simulink model "vasastaden_sort"  (Simulink 5.0)
settings: Solver=FixedStepDiscrete  SolverMode=SingleTasking  StartTime=0  StopTime=Q  FixedStep=1  RelTol=1e-3
values from neighbouring files (symbols this model uses):
  andpt = 1/3    (= 0.333333333333)    [constants_trafik.m]
  andt = 0.1    [constants_trafik.m]
  baseflow = str2num(get(HH, 'String'))    [inputs.m]
  baseflow2 = 0    [areas2.m]
  delayinit = [zeros(1,nr_ex_H2O)]    [constants_trafik.m]
  fast = 0.7    [constants_trafik.m]
  fkmday = in_fkmday    [areas.m]
  fkmday2 = 32067    [areas2.m]
  init_init = 4*3600    (= 14400)    [areas.m]
  init_time = 5    [areas.m]
  K2 = 0.03    [areas2.m]
  nhv = in_nhv/100    [areas.m]
  nhv2 = 5/100    (= 0.05)    [areas2.m]
  nr_ex_H2O = totnr-1    (= 20)    [Prep.m]
  numberOfPersons = in_numberOfPersons    [Prep.m]
  numberOfPersons2 = 5115    [areas2.m]
  othera = in_otherarea    [areas.m]
  othera2 = 42282    [areas2.m]
  othermax = drydepmax*othera    [constants_trafik.m]
  othermax2 = drydepmax*othera2    [areas2.m]
  redu = 0.8    [areas.m]
  roada = in_roads    [areas.m]
  roada2 = 95962    [areas2.m]
  roadaccmax = dryper*24*sph*fast*(p_tyrewear+p_roadwear+p_exhaust+p_breakwear+p_drydep+p_corrZn+p_oildischarge+p_catalyst)    [constants_trafik.m]
  roadaccmax2 = dryper*24*sph*fast*(p_tyrewear2+p_roadwear2+p_exhaust2+p_breakwear2+p_drydep2+p_corrZn2+p_oildischarge2+p_catalyst2)    [areas2.m]
  roadkm = 67e9    (= 67000000000)    [constants_trafik.m]
  roadrunpart = 1    [constants_trafik.m]
  roadwear = 130000    [constants_trafik.m]
  roadZna = in_part_roadZna/100*roada    [areas.m]
  roadZna2 = 2/100*roada2    (= 1919.24)    [areas2.m]
  roofa = in_roofs    [areas.m]
  roofa2 = 92958    [areas2.m]
  RoofCua = in_part_roofCua/100*roofa/cos(15*pi/180)    [areas.m]
  RoofCua2 = 6.9/100*roofa2/cos(15*pi/180)    [areas2.m]
  roofmax = (Znroofmax*RoofZna+Curoofmax*RoofCua)*roofrunpart+drydepmax*roofa    [constants_trafik.m]
  roofmax2 = (Znroofmax*RoofZna2+Curoofmax*RoofCua2)*roofrunpart+drydepmax*roofa2    [areas2.m]
  roofrunpart = 0.7    [constants_trafik.m]
  RoofZna = in_part_roofZna/100*roofa/cos(15*pi/180)    [areas.m]
  RoofZna2 = 6.4/100*roofa2/cos(15*pi/180)    [areas2.m]
  sec_per_ts = in_sec_per_ts    [Prep.m]
  sph = 3600/sec_per_ts    [Prep.m]
  tota = in_tota    [areas.m]
  totnr = 21    [Prep.m]
  tyrewear = 9000    [constants_trafik.m]
  wetdep = [sum(s_wetdep(:,i))]*tota*trans1    [polldistr_gr.m]
  yearly_rain = 1    [Callback_simulate.m]    (also in SEWSYS_fig.m)
undefined symbols (not defined in the file or in its folder): BDT, BODofVS, brakep, catalystp, Curoofp, Drainage, drydep, exhp, Faeces, Industry, K, K2r, oilp, ProcSS_bio, ProcSS_chem, ProcSS_presed, ProcSS_sand, ProcSS_screen, roadp, sani, spBiooxidBod, spBiored, spCcontent, spChemFe, spChemicalPart, spCODBOD, spDenSS, spHeavym, spHjust, spN2ONpurEmitted, spNemitted, spNitrif, spNpur, spOcontent, spPBound, spPout, spPout1, spVSofSS, SSred_bio, SSred_chem, SSred_presed, SSred_sand, SSred_screen, SStoWater, stormw, tyrep, Urine, VSofSS_sand, VSofSS_screen, Znroofp
libraries: SEWSYS_library x1
(part 2 of 3)

== system vasastaden_sort/Sewage plant/Pre-sedimentation/Separation/3-6 ==
  in_1 : Inport  Orientation=down
  "in_2 " : Inport  Orientation=down  Port=2
  Ground1 : Ground  Orientation=down
  Mux : Mux  Orientation=down
  N-tot : MATLABFcn  Orientation=down  MATLABFcn=(u(1)-u(2)-u(3))*SSred_presed  OutputDimensions=1
  NH4 : Product  Orientation=down  SaturateOnIntegerOverflow=on  InputSameDT=on
  "NH4 " : Fcn  Orientation=down  Expr=u(2)
  NH5 : Product  Orientation=down  SaturateOnIntegerOverflow=on  InputSameDT=on
  NO3 : Fcn  Orientation=down  Expr=u(3)
  Sum : Sum  Orientation=down  Inputs=+++  SaturateOnIntegerOverflow=on  InputSameDT=on
  out_1 : Outport  Orientation=down  InitialOutput=0
  wires:
  NH4/1 -> Mux/2, Sum/2
  in_1/1 -> NH5/1, NH4/1
  Mux/1 -> out_1/1
  N-tot/1 -> Sum/1
  Sum/1 -> Mux/1
  "NH4 "/1 -> NH4/2
  NO3/1 -> NH5/2
  "in_2 "/1 -> NO3/1, "NH4 "/1, N-tot/1
  NH5/1 -> Sum/3, Mux/3
  Ground1/1 -> Mux/4

== system vasastaden_sort/Sewage plant/Pre-sedimentation/Separation/if u>0 then 1/u else 0 ==
  note: if u<=0, 0, else 1/u, end
  in_1 : Inport  Orientation=left
  Constant : Constant  Orientation=left  Value=0
  Constant1 : Constant  Orientation=left
  Switch : Switch  Orientation=left  SaturateOnIntegerOverflow=on  InputSameDT=on
  Switch1 : Switch  Orientation=left  SaturateOnIntegerOverflow=on  InputSameDT=on
  inv. : Fcn  Orientation=left  Expr=1/u
  neg : Gain  Orientation=left  Gain=-1  SaturateOnIntegerOverflow=on
  neg1 : Gain  Orientation=left  Gain=-1  SaturateOnIntegerOverflow=on
  out_1 : Outport  Orientation=left  InitialOutput=0
  wires:
  Constant/1 -> Switch/1
  neg/1 -> Switch/2
  Switch/1 -> out_1/1
  inv./1 -> Switch/3
  Switch1/1 -> inv./1
  neg1/1 -> Switch1/2
  Constant1/1 -> Switch1/1
  in_1/1 -> neg/1, neg1/1, Switch1/3

== system vasastaden_sort/Sewage plant/Pre-sedimentation/spVSofSS/if u>0 then 1/u else 0 ==
  note: if u<=0, 0, else 1/u, end
  in_1 : Inport  Orientation=left
  Constant : Constant  Orientation=left  Value=0
  Constant1 : Constant  Orientation=left
  Switch : Switch  Orientation=left  SaturateOnIntegerOverflow=on  InputSameDT=on
  Switch1 : Switch  Orientation=left  SaturateOnIntegerOverflow=on  InputSameDT=on
  inv. : Fcn  Orientation=left  Expr=1/u
  neg : Gain  Orientation=left  Gain=-1  SaturateOnIntegerOverflow=on
  neg1 : Gain  Orientation=left  Gain=-1  SaturateOnIntegerOverflow=on
  out_1 : Outport  Orientation=left  InitialOutput=0
  wires:
  inv./1 -> Switch/3
  Constant/1 -> Switch/1
  neg/1 -> Switch/2
  Switch1/1 -> inv./1
  Switch/1 -> out_1/1
  neg1/1 -> Switch1/2
  Constant1/1 -> Switch1/1
  in_1/1 -> neg/1, neg1/1, Switch1/3

== system vasastaden_sort/Sewage plant/Sandpit/Separation/3-6 ==
  in_1 : Inport  Orientation=down
  "in_2 " : Inport  Orientation=down  Port=2
  Ground2 : Ground  Orientation=down
  Mux : Mux  Orientation=down
  N-tot : MATLABFcn  Orientation=down  MATLABFcn=(u(1)-u(2)-u(3))*SSred_sand  OutputDimensions=1
  NH4 : Product  Orientation=down  SaturateOnIntegerOverflow=on  InputSameDT=on
  "NH4 " : Fcn  Orientation=down  Expr=u(2)
  NH5 : Product  Orientation=down  SaturateOnIntegerOverflow=on  InputSameDT=on
  NO3 : Fcn  Orientation=down  Expr=u(3)
  Sum : Sum  Orientation=down  Inputs=+++  SaturateOnIntegerOverflow=on  InputSameDT=on
  out_1 : Outport  Orientation=down  InitialOutput=0
  wires:
  Ground2/1 -> Mux/4
  NH5/1 -> Mux/3, Sum/3
  "in_2 "/1 -> N-tot/1, "NH4 "/1, NO3/1
  NO3/1 -> NH5/2
  "NH4 "/1 -> NH4/2
  Sum/1 -> Mux/1
  N-tot/1 -> Sum/1
  Mux/1 -> out_1/1
  in_1/1 -> NH4/1, NH5/1
  NH4/1 -> Sum/2, Mux/2

== system vasastaden_sort/Sewage plant/Sandpit/Separation/if u>0 then 1/u else 0 ==
  note: if u<=0, 0, else 1/u, end
  in_1 : Inport  Orientation=left
  Constant : Constant  Orientation=left  Value=0
  Constant1 : Constant  Orientation=left
  Switch : Switch  Orientation=left  SaturateOnIntegerOverflow=on  InputSameDT=on
  Switch1 : Switch  Orientation=left  SaturateOnIntegerOverflow=on  InputSameDT=on
  inv. : Fcn  Orientation=left  Expr=1/u
  neg : Gain  Orientation=left  Gain=-1  SaturateOnIntegerOverflow=on
  neg1 : Gain  Orientation=left  Gain=-1  SaturateOnIntegerOverflow=on
  out_1 : Outport  Orientation=left  InitialOutput=0
  wires:
  Switch/1 -> out_1/1
  neg/1 -> Switch/2
  Constant/1 -> Switch/1
  inv./1 -> Switch/3
  Switch1/1 -> inv./1
  neg1/1 -> Switch1/2
  Constant1/1 -> Switch1/1
  in_1/1 -> neg/1, neg1/1, Switch1/3

== system vasastaden_sort/Sewage plant/Screen/Separation/3-6 ==
  in_1 : Inport  Orientation=down
  "in_2 " : Inport  Orientation=down  Port=2
  Ground : Ground  Orientation=down
  Mux : Mux  Orientation=down
  N-tot : MATLABFcn  Orientation=down  MATLABFcn=(u(1)-u(2)-u(3))*SSred_screen  OutputDimensions=1
  NH4 : Product  Orientation=down  SaturateOnIntegerOverflow=on  InputSameDT=on
  "NH4 " : Fcn  Orientation=down  Expr=u(2)
  NH5 : Product  Orientation=down  SaturateOnIntegerOverflow=on  InputSameDT=on
  NO3 : Fcn  Orientation=down  Expr=u(3)
  Sum : Sum  Orientation=down  Inputs=+++  SaturateOnIntegerOverflow=on  InputSameDT=on
  out_1 : Outport  Orientation=down  InitialOutput=0
  wires:
  NH4/1 -> Mux/2, Sum/2
  in_1/1 -> NH5/1, NH4/1
  Mux/1 -> out_1/1
  N-tot/1 -> Sum/1
  Sum/1 -> Mux/1
  "NH4 "/1 -> NH4/2
  NO3/1 -> NH5/2
  "in_2 "/1 -> NO3/1, "NH4 "/1, N-tot/1
  NH5/1 -> Sum/3, Mux/3
  Ground/1 -> Mux/4

== system vasastaden_sort/Sewage plant/Screen/Separation/if u>0 then 1/u else 0 ==
  note: if u<=0, 0, else 1/u, end
  in_1 : Inport  Orientation=left
  Constant : Constant  Orientation=left  Value=0
  Constant1 : Constant  Orientation=left
  Switch : Switch  Orientation=left  SaturateOnIntegerOverflow=on  InputSameDT=on
  Switch1 : Switch  Orientation=left  SaturateOnIntegerOverflow=on  InputSameDT=on
  inv. : Fcn  Orientation=left  Expr=1/u
  neg : Gain  Orientation=left  Gain=-1  SaturateOnIntegerOverflow=on
  neg1 : Gain  Orientation=left  Gain=-1  SaturateOnIntegerOverflow=on
  out_1 : Outport  Orientation=left  InitialOutput=0
  wires:
  Constant/1 -> Switch/1
  neg/1 -> Switch/2
  Switch/1 -> out_1/1
  inv./1 -> Switch/3
  Switch1/1 -> inv./1
  neg1/1 -> Switch1/2
  Constant1/1 -> Switch1/1
  in_1/1 -> neg/1, neg1/1, Switch1/3

== system vasastaden_sort/Separate Sewer System  (36)/Sanitary Wastewater/Sanitary wastewater/Household/Greywater ==
  "Greywater " : Constant  Value=BDT
  Out : Outport
  wires:
  "Greywater "/1 -> Out/1

== system vasastaden_sort/Separate Sewer System  (36)/Sanitary Wastewater/Sanitary wastewater/Household/Toilet ==
  "Faeces & paper " : Constant  Value=Faeces
  Sum : Sum  SaturateOnIntegerOverflow=on  InputSameDT=on
  "Urine " : Constant  Value=Urine
  Out : Outport
  wires:
  Sum/1 -> Out/1
  "Urine "/1 -> Sum/1
  "Faeces & paper "/1 -> Sum/2

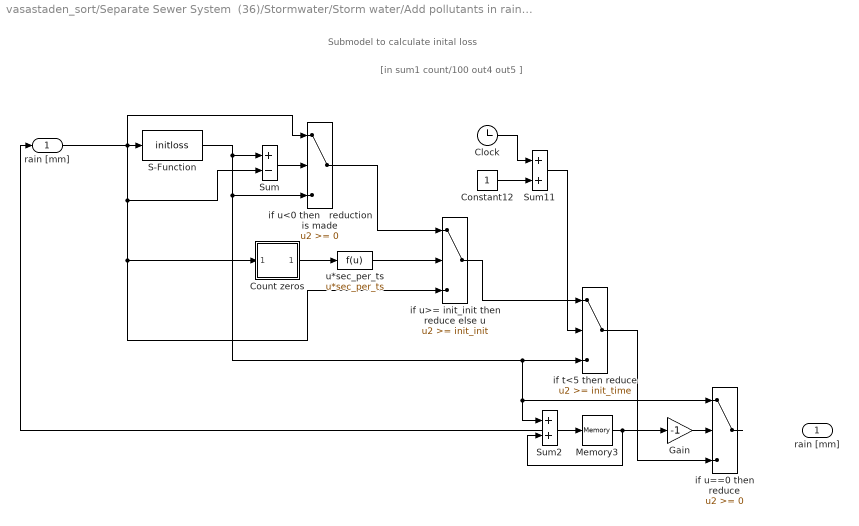
== system vasastaden_sort/Separate Sewer System  (36)/Stormwater/Storm water/Add pollutants in rain/Initial loss ==
  note: Submodel to calculate inital loss
  note: [in sum1 count/100 out4 out5 ]
  rain [mm] : Inport
  Clock : Clock
      settings: Decimation=10
  Constant12 : Constant
  Count zeros : Subsystem
  Gain : Gain  Gain=-1  SaturateOnIntegerOverflow=on
  Memory3 : Memory
  S-Function : S-Function  FunctionName=initloss  Parameters=init
  Sum : Sum  Inputs=+-  SaturateOnIntegerOverflow=on  InputSameDT=on
  Sum11 : Sum  SaturateOnIntegerOverflow=on  InputSameDT=on
  Sum2 : Sum  SaturateOnIntegerOverflow=on  InputSameDT=on
  if t<5 then reduce : Switch  Threshold=init_time  SaturateOnIntegerOverflow=on  InputSameDT=on
  if u<0 then   reduction is made : Switch  SaturateOnIntegerOverflow=on  InputSameDT=on
  if u==0 then reduce : Switch  SaturateOnIntegerOverflow=on  InputSameDT=on
  if u>= init_init then reduce else u : Switch  Threshold=init_init  SaturateOnIntegerOverflow=on  InputSameDT=on
  u*sec_per_ts : Fcn  Expr=u*sec_per_ts
  rain [mm] : Outport
  wires:
  S-Function/1 -> Sum/1, if u<0 then   reduction is made/3, if t<5 then reduce/3, if u==0 then reduce/1, Sum2/1
  Sum11/1 -> if t<5 then reduce/2
  Sum/1 -> if u<0 then   reduction is made/2
  if u<0 then   reduction is made/1 -> if u>= init_init then reduce else u/1
  rain [mm]/1 -> Count zeros/1(In1), if u>= init_init then reduce else u/3, Sum/2, S-Function/1, if u<0 then   reduction is made/1
  Count zeros/1(Out1) -> u*sec_per_ts/1
  u*sec_per_ts/1 -> if u>= init_init then reduce else u/2
  Clock/1 -> Sum11/1
  Constant12/1 -> Sum11/2
  Gain/1 -> if u==0 then reduce/2
  if u==0 then reduce/1 -> rain [mm]/1
  Memory3/1 -> Gain/1, Sum2/2
  Sum2/1 -> Memory3/1
  if u>= init_init then reduce else u/1 -> if t<5 then reduce/1
  if t<5 then reduce/1 -> if u==0 then reduce/3

== system vasastaden_sort/Separate Sewer System  (36)/Stormwater/Storm water/Add pollutants in rain/wet deposition ==
  rain [mm] : Inport
  Mux : Mux  Inputs=2
  Product1 : Product  SaturateOnIntegerOverflow=on  InputSameDT=on
  Product2 : Product  Inputs=*/  SaturateOnIntegerOverflow=on  InputSameDT=on
  To Workspace6 : ToWorkspace  VariableName=s_wetdep2  SampleTime=-1  SaveFormat=Array
  rain mm/yr : Constant  Value=yearly_rain
  wet deposition ug/m2*yr : Constant  Value=wetdep
  rain [mm] pollutants [ug/m2] : Outport
  wires:
  rain [mm]/1 -> Product1/1, Mux/1
  Product2/1 -> Product1/2
  wet deposition ug/m2*yr/1 -> Product2/1
  rain mm/yr/1 -> Product2/2
  Product1/1 -> Mux/2
  Mux/1 -> rain [mm] pollutants [ug/m2]/1, To Workspace6/1

== system vasastaden_sort/Separate Sewer System  (36)/Stormwater/Storm water/Rain -> Stormwater/other surfaces ==
  rain[mm] pollutants [ug/m2] : Inport
  Demux2 : Demux  Outputs=[1 -1]
  Mux2 : Mux  Inputs=2
  Product1 : Product  SaturateOnIntegerOverflow=on  InputSameDT=on
  Sum : Sum  Inputs=|++  SaturateOnIntegerOverflow=on  InputSameDT=on
  To Workspace7 : ToWorkspace  VariableName=s_other2  SampleTime=-1  SaveFormat=Array
  ackumulation and wash-off : Subsystem
  area [m2] : Constant  Value=othera2
  dry deposition : Subsystem
  rain on other surfaces : Subsystem
  ug - g : Gain  Gain=0.000001  SaturateOnIntegerOverflow=on
  rain[m3] pollutants [g] : Outport
  wires:
  rain[mm] pollutants [ug/m2]/1 -> Demux2/1
  Mux2/1 -> rain[m3] pollutants [g]/1
  area [m2]/1 -> Product1/2
  Demux2/2 -> Product1/1
  Demux2/1 -> ackumulation and wash-off/1(rain [mm]), rain on other surfaces/1(rain [mm])
  dry deposition/1(pollutants [ug]) -> ackumulation and wash-off/2(pollutant [ug])
  Product1/1 -> Sum/2
  rain on other surfaces/1(rain [m3]) -> Mux2/1
  Sum/1 -> ug - g/1
  ug - g/1 -> Mux2/2
  ackumulation and wash-off/1(pollutants [ug]) -> Sum/1, To Workspace7/1

== system vasastaden_sort/Separate Sewer System  (36)/Stormwater/Storm water/Rain -> Stormwater/road surfaces ==
  rain [mm] pollutants [ug/m2] : Inport
  Demux1 : Demux  Outputs=[1 -1]
  Mux3 : Mux  Inputs=2
  Sum1 : Sum  Inputs=|++  SaturateOnIntegerOverflow=on  InputSameDT=on
  To Workspace7 : ToWorkspace  VariableName=s_road2  SampleTime=-1  SaveFormat=Array
  accumulation and wash-off : Subsystem
  pollutants on roads : Subsystem
  rain on road : Subsystem
  ug - g : Gain  Gain=0.000001  SaturateOnIntegerOverflow=on
  rain[m3] pollutants [g] : Outport
  wires:
  rain on road/1(rain [m3]) -> Mux3/1
  accumulation and wash-off/1(rain [mm]1) -> rain on road/1(rain [mm])
  Demux1/2 -> rain on road/2(pollutants [ug/m2])
  Demux1/1 -> accumulation and wash-off/1(rain [mm])
  rain [mm] pollutants [ug/m2]/1 -> Demux1/1
  Mux3/1 -> rain[m3] pollutants [g]/1
  rain on road/2(pollutants [ug]) -> Sum1/1
  accumulation and wash-off/2(pollutants [ug]) -> Sum1/2, To Workspace7/1
  Sum1/1 -> ug - g/1
  ug - g/1 -> Mux3/2
  pollutants on roads/1(pollutants[ ug]) -> accumulation and wash-off/2(pollutant [ug])

== system vasastaden_sort/Separate Sewer System  (36)/Stormwater/Storm water/Rain -> Stormwater/roofs ==
  note: Accumulates pollutants over time. Washes out during rain.
  rain [mm]  pollutants[ug/m2] : Inport
  Demux : Demux  Outputs=[1 -1]
  Mux : Mux  Inputs=2
  Pollutants on roofs : Subsystem
  Product : Product  SaturateOnIntegerOverflow=on  InputSameDT=on
  Sum : Sum  Inputs=|++  SaturateOnIntegerOverflow=on  InputSameDT=on
  To Workspace7 : ToWorkspace  VariableName=s_roof2  SampleTime=-1  SaveFormat=Array
  ackumulation and wash-off : Subsystem
  area [m2] : Constant  Value=roofa2
  rain on roof surfaces : Subsystem
  ug - g : Gain  Gain=0.000001  SaturateOnIntegerOverflow=on
  rain[m3] pollutants [g] : Outport
  wires:
  Mux/1 -> rain[m3] pollutants [g]/1
  area [m2]/1 -> Product/2
  Demux/2 -> Product/1
  rain on roof surfaces/1(rain [m3]) -> Mux/1
  rain [mm]  pollutants[ug/m2]/1 -> Demux/1
  Product/1 -> Sum/2
  Sum/1 -> ug - g/1
  ug - g/1 -> Mux/2
  Demux/1 -> rain on roof surfaces/1(rain [mm]), ackumulation and wash-off/1(rain [mm])
  ackumulation and wash-off/1(pollutants [ug]) -> Sum/1, To Workspace7/1
  Pollutants on roofs/1(pollutants [ug]) -> ackumulation and wash-off/2(pollutant [ug])

== system vasastaden_sort/Separate Sewer System  (36)/Stormwater/Storm water/Runoff/Make per second ==
  In1 : Inport
  Demux : Demux  Outputs=[1 -1]
  Mux1 : Mux  Inputs=2
  g - g/s : Gain  Gain=1/sec_per_ts  SaturateOnIntegerOverflow=on
  m3 - m3/s : Gain  Gain=1/sec_per_ts  SaturateOnIntegerOverflow=on
  Out1 : Outport
  wires:
  In1/1 -> Demux/1
  Mux1/1 -> Out1/1
  Demux/1 -> m3 - m3/s/1
  m3 - m3/s/1 -> Mux1/1
  Demux/2 -> g - g/s/1
  g - g/s/1 -> Mux1/2

== system vasastaden_sort/Separate Sewer System  (36)/Stormwater/Storm water/Runoff/Subsystem1 ==
  In1 : Inport
  Gain : Gain  Gain=sec_per_ts  SaturateOnIntegerOverflow=on
  Qut : Fcn  Expr=(roofa2+othera2)*K2*u^(5/3)
  Sum : Sum  SaturateOnIntegerOverflow=on  InputSameDT=on
  Sum1 : Sum  Inputs=+-  SaturateOnIntegerOverflow=on  InputSameDT=on
  Sum2 : Sum  SaturateOnIntegerOverflow=on  InputSameDT=on
  Unit Delay1 : UnitDelay  Orientation=left
  Unit Delay2 : UnitDelay
  if u>0 then u else 1 : Subsystem
      mask Display: disp('1/u')
  y : Fcn  Expr=u/(roofa2+othera2)
  yprim : Fcn  Expr=u*sec_per_ts/(roofa2+othera2)/3
  Out1 : Outport
  wires:
  Qut/1 -> Sum1/2, Out1/1
  Unit Delay1/1 -> Sum2/2
  Sum2/1 -> Unit Delay1/1, y/1
  Gain/1 -> Sum2/1
  Sum1/1 -> Gain/1
  y/1 -> if u>0 then u else 1/1(in_1)
  yprim/1 -> Sum/1
  Sum/1 -> Qut/1
  if u>0 then u else 1/1(out_1) -> Unit Delay2/1
  Unit Delay2/1 -> Sum/2
  In1/1 -> Sum1/1, yprim/1

== system vasastaden_sort/Separate Sewer System  (36)/Stormwater/Storm water/Runoff (roads)/Make per second ==
  In1 : Inport
  Demux : Demux  Outputs=[1 -1]
  Mux1 : Mux  Inputs=2
  g - g/s : Gain  Gain=1/sec_per_ts  SaturateOnIntegerOverflow=on
  m3 - m3/s : Gain  Gain=1/sec_per_ts  SaturateOnIntegerOverflow=on
  Out1 : Outport
  wires:
  g - g/s/1 -> Mux1/2
  Demux/2 -> g - g/s/1
  m3 - m3/s/1 -> Mux1/1
  Demux/1 -> m3 - m3/s/1
  Mux1/1 -> Out1/1
  In1/1 -> Demux/1

== system vasastaden_sort/Separate Sewer System  (36)/Stormwater/Storm water/Runoff (roads)/Subsystem1 ==
  In1 : Inport
  Gain : Gain  Gain=sec_per_ts  SaturateOnIntegerOverflow=on
  Qut : Fcn  Expr=roada2*K2r*u^(5/3)
  Sum : Sum  SaturateOnIntegerOverflow=on  InputSameDT=on
  Sum1 : Sum  Inputs=+-  SaturateOnIntegerOverflow=on  InputSameDT=on
  Sum2 : Sum  SaturateOnIntegerOverflow=on  InputSameDT=on
  Unit Delay1 : UnitDelay  Orientation=left
  Unit Delay2 : UnitDelay
  if u>0 then u else 1 : Subsystem
      mask Display: disp('1/u')
  y : Fcn  Expr=u/roada2
  yprim : Fcn  Expr=u*sec_per_ts/roada2/3
  Out1 : Outport
  wires:
  In1/1 -> yprim/1, Sum1/1
  Unit Delay2/1 -> Sum/2
  if u>0 then u else 1/1(out_1) -> Unit Delay2/1
  Sum/1 -> Qut/1
  yprim/1 -> Sum/1
  y/1 -> if u>0 then u else 1/1(in_1)
  Sum1/1 -> Gain/1
  Gain/1 -> Sum2/1
  Sum2/1 -> y/1, Unit Delay1/1
  Unit Delay1/1 -> Sum2/2
  Qut/1 -> Out1/1, Sum1/2

== system vasastaden_sort/Separate Sewer System  (1245)/Sanitary Wastewater/Sanitary wastewater/Household/Greywater ==
  "Greywater " : Constant  Value=BDT
  To Workspace6 : ToWorkspace  VariableName=s_bdt  SampleTime=-1  SaveFormat=Array
      settings: MaxDataPoints=1
  Out : Outport
  wires:
  "Greywater "/1 -> To Workspace6/1, Out/1

== system vasastaden_sort/Separate Sewer System  (1245)/Sanitary Wastewater/Sanitary wastewater/Household/Toilet ==
  "Faeces & paper " : Constant  Value=Faeces
  Sum : Sum  SaturateOnIntegerOverflow=on  InputSameDT=on
  To Workspace6 : ToWorkspace  VariableName=s_urine  SampleTime=-1  SaveFormat=Array
      settings: MaxDataPoints=1
  To Workspace7 : ToWorkspace  VariableName=s_faeces  SampleTime=-1  SaveFormat=Array
      settings: MaxDataPoints=1
  "Urine " : Constant  Value=Urine
  Out : Outport
  wires:
  "Faeces & paper "/1 -> To Workspace7/1, Sum/2
  "Urine "/1 -> To Workspace6/1, Sum/1
  Sum/1 -> Out/1

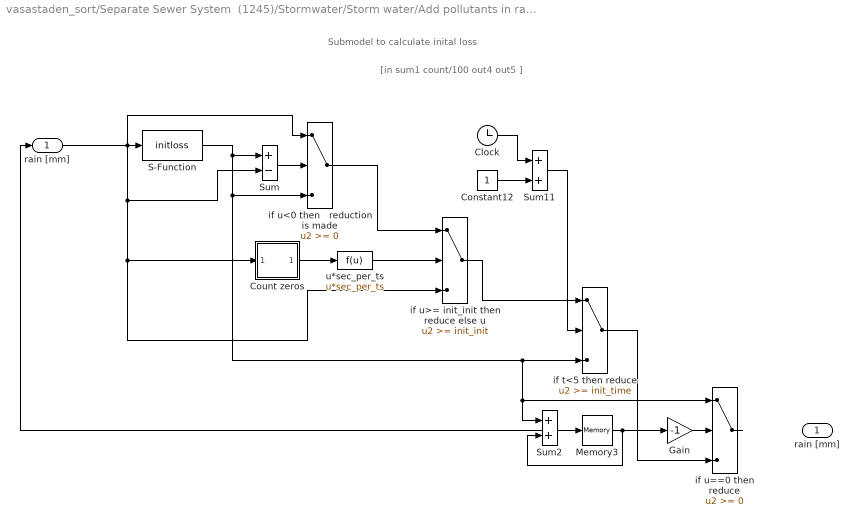
== system vasastaden_sort/Separate Sewer System  (1245)/Stormwater/Storm water/Add pollutants in rain/Initial loss ==
  note: [in sum1 count/100 out4 out5 ]
  note: Submodel to calculate inital loss
  rain [mm] : Inport
  Clock : Clock
      settings: Decimation=10
  Constant12 : Constant
  Count zeros : Subsystem
  Gain : Gain  Gain=-1  SaturateOnIntegerOverflow=on
  Memory3 : Memory
  S-Function : S-Function  FunctionName=initloss  Parameters=init
  Sum : Sum  Inputs=+-  SaturateOnIntegerOverflow=on  InputSameDT=on
  Sum11 : Sum  SaturateOnIntegerOverflow=on  InputSameDT=on
  Sum2 : Sum  SaturateOnIntegerOverflow=on  InputSameDT=on
  if t<5 then reduce : Switch  Threshold=init_time  SaturateOnIntegerOverflow=on  InputSameDT=on
  if u<0 then   reduction is made : Switch  SaturateOnIntegerOverflow=on  InputSameDT=on
  if u==0 then reduce : Switch  SaturateOnIntegerOverflow=on  InputSameDT=on
  if u>= init_init then reduce else u : Switch  Threshold=init_init  SaturateOnIntegerOverflow=on  InputSameDT=on
  u*sec_per_ts : Fcn  Expr=u*sec_per_ts
  rain [mm] : Outport
  wires:
  if t<5 then reduce/1 -> if u==0 then reduce/3
  if u>= init_init then reduce else u/1 -> if t<5 then reduce/1
  Sum2/1 -> Memory3/1
  Memory3/1 -> Gain/1, Sum2/2
  if u==0 then reduce/1 -> rain [mm]/1
  Gain/1 -> if u==0 then reduce/2
  Constant12/1 -> Sum11/2
  Clock/1 -> Sum11/1
  u*sec_per_ts/1 -> if u>= init_init then reduce else u/2
  Count zeros/1(Out1) -> u*sec_per_ts/1
  rain [mm]/1 -> if u<0 then   reduction is made/1, S-Function/1, Sum/2, if u>= init_init then reduce else u/3, Count zeros/1(In1)
  if u<0 then   reduction is made/1 -> if u>= init_init then reduce else u/1
  Sum/1 -> if u<0 then   reduction is made/2
  Sum11/1 -> if t<5 then reduce/2
  S-Function/1 -> Sum2/1, if u==0 then reduce/1, if t<5 then reduce/3, if u<0 then   reduction is made/3, Sum/1

== system vasastaden_sort/Separate Sewer System  (1245)/Stormwater/Storm water/Add pollutants in rain/wet deposition ==
  rain [mm] : Inport
  Mux : Mux  Inputs=2
  Product1 : Product  SaturateOnIntegerOverflow=on  InputSameDT=on
  Product2 : Product  Inputs=*/  SaturateOnIntegerOverflow=on  InputSameDT=on
  To Workspace6 : ToWorkspace  VariableName=s_wetdep  SampleTime=-1  SaveFormat=Array
  rain mm/yr : Constant  Value=yearly_rain
  wet deposition ug/m2*yr : Constant  Value=wetdep
  rain [mm] pollutants [ug/m2] : Outport
  wires:
  Mux/1 -> To Workspace6/1, rain [mm] pollutants [ug/m2]/1
  Product1/1 -> Mux/2
  rain mm/yr/1 -> Product2/2
  wet deposition ug/m2*yr/1 -> Product2/1
  Product2/1 -> Product1/2
  rain [mm]/1 -> Mux/1, Product1/1

== system vasastaden_sort/Separate Sewer System  (1245)/Stormwater/Storm water/Rain -> Stormwater/other surfaces ==
  rain[mm] pollutants [ug/m2] : Inport
  Demux2 : Demux  Outputs=[1 -1]
  Mux2 : Mux  Inputs=2
  Product1 : Product  SaturateOnIntegerOverflow=on  InputSameDT=on
  Sum : Sum  Inputs=|++  SaturateOnIntegerOverflow=on  InputSameDT=on
  To Workspace7 : ToWorkspace  VariableName=s_other  SampleTime=-1  SaveFormat=Array
  ackumulation and wash-off : Subsystem
  area [m2] : Constant  Value=othera
  dry deposition : Subsystem
  rain on other surfaces : Subsystem
  ug - g : Gain  Gain=0.000001  SaturateOnIntegerOverflow=on
  rain[m3] pollutants [g] : Outport
  wires:
  ackumulation and wash-off/1(pollutants [ug]) -> To Workspace7/1, Sum/1
  ug - g/1 -> Mux2/2
  Sum/1 -> ug - g/1
  rain on other surfaces/1(rain [m3]) -> Mux2/1
  Product1/1 -> Sum/2
  dry deposition/1(pollutants [ug]) -> ackumulation and wash-off/2(pollutant [ug])
  Demux2/1 -> rain on other surfaces/1(rain [mm]), ackumulation and wash-off/1(rain [mm])
  Demux2/2 -> Product1/1
  area [m2]/1 -> Product1/2
  Mux2/1 -> rain[m3] pollutants [g]/1
  rain[mm] pollutants [ug/m2]/1 -> Demux2/1

== system vasastaden_sort/Separate Sewer System  (1245)/Stormwater/Storm water/Rain -> Stormwater/road surfaces ==
  rain [mm] pollutants [ug/m2] : Inport
  Demux1 : Demux  Outputs=[1 -1]
  Mux3 : Mux  Inputs=2
  Sum1 : Sum  Inputs=|++  SaturateOnIntegerOverflow=on  InputSameDT=on
  To Workspace7 : ToWorkspace  VariableName=s_road  SampleTime=-1  SaveFormat=Array
  accumulation and wash-off : Subsystem
  pollutants on roads : Subsystem
  rain on road : Subsystem
  ug - g : Gain  Gain=0.000001  SaturateOnIntegerOverflow=on
  rain[m3] pollutants [g] : Outport
  wires:
  pollutants on roads/1(pollutants[ ug]) -> accumulation and wash-off/2(pollutant [ug])
  ug - g/1 -> Mux3/2
  Sum1/1 -> ug - g/1
  accumulation and wash-off/2(pollutants [ug]) -> To Workspace7/1, Sum1/2
  rain on road/2(pollutants [ug]) -> Sum1/1
  Mux3/1 -> rain[m3] pollutants [g]/1
  rain [mm] pollutants [ug/m2]/1 -> Demux1/1
  Demux1/1 -> accumulation and wash-off/1(rain [mm])
  Demux1/2 -> rain on road/2(pollutants [ug/m2])
  accumulation and wash-off/1(rain [mm]1) -> rain on road/1(rain [mm])
  rain on road/1(rain [m3]) -> Mux3/1

== system vasastaden_sort/Separate Sewer System  (1245)/Stormwater/Storm water/Rain -> Stormwater/roofs ==
  note: Accumulates pollutants over time. Washes out during rain.
  rain [mm]  pollutants[ug/m2] : Inport
  Demux : Demux  Outputs=[1 -1]
  Mux : Mux  Inputs=2
  Pollutants on roofs : Subsystem
  Product : Product  SaturateOnIntegerOverflow=on  InputSameDT=on
  Sum : Sum  Inputs=|++  SaturateOnIntegerOverflow=on  InputSameDT=on
  To Workspace7 : ToWorkspace  VariableName=s_roof  SampleTime=-1  SaveFormat=Array
  ackumulation and wash-off : Subsystem
  area [m2] : Constant  Value=roofa
  rain on roof surfaces : Subsystem
  ug - g : Gain  Gain=0.000001  SaturateOnIntegerOverflow=on
  rain[m3] pollutants [g] : Outport
  wires:
  Pollutants on roofs/1(pollutants [ug]) -> ackumulation and wash-off/2(pollutant [ug])
  ackumulation and wash-off/1(pollutants [ug]) -> To Workspace7/1, Sum/1
  Demux/1 -> ackumulation and wash-off/1(rain [mm]), rain on roof surfaces/1(rain [mm])
  ug - g/1 -> Mux/2
  Sum/1 -> ug - g/1
  Product/1 -> Sum/2
  rain [mm]  pollutants[ug/m2]/1 -> Demux/1
  rain on roof surfaces/1(rain [m3]) -> Mux/1
  Demux/2 -> Product/1
  area [m2]/1 -> Product/2
  Mux/1 -> rain[m3] pollutants [g]/1

== system vasastaden_sort/Separate Sewer System  (1245)/Stormwater/Storm water/Runoff/Make per second ==
  In1 : Inport
  Demux : Demux  Outputs=[1 -1]
  Mux1 : Mux  Inputs=2
  g - g/s : Gain  Gain=1/sec_per_ts  SaturateOnIntegerOverflow=on
  m3 - m3/s : Gain  Gain=1/sec_per_ts  SaturateOnIntegerOverflow=on
  Out1 : Outport
  wires:
  g - g/s/1 -> Mux1/2
  Demux/2 -> g - g/s/1
  m3 - m3/s/1 -> Mux1/1
  Demux/1 -> m3 - m3/s/1
  Mux1/1 -> Out1/1
  In1/1 -> Demux/1

== system vasastaden_sort/Separate Sewer System  (1245)/Stormwater/Storm water/Runoff/Subsystem1 ==
  In1 : Inport
  Gain : Gain  Gain=sec_per_ts  SaturateOnIntegerOverflow=on
  Qut : Fcn  Expr=tota*K*u^(5/3)
  Sum : Sum  SaturateOnIntegerOverflow=on  InputSameDT=on
  Sum1 : Sum  Inputs=+-  SaturateOnIntegerOverflow=on  InputSameDT=on
  Sum2 : Sum  SaturateOnIntegerOverflow=on  InputSameDT=on
  Unit Delay1 : UnitDelay  Orientation=left
  Unit Delay2 : UnitDelay
  if u>0 then u else 1 : Subsystem
      mask Display: disp('1/u')
  y : Fcn  Expr=u/tota
  yprim : Fcn  Expr=u*sec_per_ts/tota/3
  Out1 : Outport
  wires:
  In1/1 -> yprim/1, Sum1/1
  Unit Delay2/1 -> Sum/2
  if u>0 then u else 1/1(out_1) -> Unit Delay2/1
  Sum/1 -> Qut/1
  yprim/1 -> Sum/1
  y/1 -> if u>0 then u else 1/1(in_1)
  Sum1/1 -> Gain/1
  Gain/1 -> Sum2/1
  Sum2/1 -> y/1, Unit Delay1/1
  Unit Delay1/1 -> Sum2/2
  Qut/1 -> Out1/1, Sum1/2

== system vasastaden_sort/Sewage plant/Biological stage/Predenitri- fication/N-org to NH4 through oxid to CO2/if u>0 then 1/u else 0 ==
  note: if u<=0, 0, else 1/u, end
  in_1 : Inport  Orientation=left
  Constant : Constant  Orientation=left  Value=0
  Constant1 : Constant  Orientation=left
  Switch : Switch  Orientation=left  SaturateOnIntegerOverflow=on  InputSameDT=on
  Switch1 : Switch  Orientation=left  SaturateOnIntegerOverflow=on  InputSameDT=on
  inv. : Fcn  Orientation=left  Expr=1/u
  neg : Gain  Orientation=left  Gain=-1  SaturateOnIntegerOverflow=on
  out_1 : Outport  Orientation=left  InitialOutput=0
  wires:
  Constant1/1 -> Switch1/1
  in_1/1 -> Switch1/3, neg/1
  neg/1 -> Switch1/2, Switch/2
  Switch1/1 -> inv./1
  Switch/1 -> out_1/1
  inv./1 -> Switch/3
  Constant/1 -> Switch/1

== system vasastaden_sort/Sewage plant/Biological stage/Predenitri- fication/NH3 emissions from  aeration to nitrification  and degration of BOD./if u>0 then 1/u else 0 ==
  note: if u<=0, 0, else 1/u, end
  in_1 : Inport  Orientation=left
  Constant : Constant  Orientation=left  Value=0
  Constant1 : Constant  Orientation=left
  Switch : Switch  Orientation=left  SaturateOnIntegerOverflow=on  InputSameDT=on
  Switch1 : Switch  Orientation=left  SaturateOnIntegerOverflow=on  InputSameDT=on
  inv. : Fcn  Orientation=left  Expr=1/u
  neg : Gain  Orientation=left  Gain=-1  SaturateOnIntegerOverflow=on
  out_1 : Outport  Orientation=left  InitialOutput=0
  wires:
  Constant1/1 -> Switch1/1
  in_1/1 -> Switch1/3, neg/1
  neg/1 -> Switch1/2, Switch/2
  Switch1/1 -> inv./1
  Switch/1 -> out_1/1
  inv./1 -> Switch/3
  Constant/1 -> Switch/1

== system vasastaden_sort/Sewage plant/Biological stage/Predenitri- fication/NH3 emissions from  aeration to nitrification  and degration of BOD./if u>0 then 1/u else 1 ==
  note: if u<=0, 0, else 1/u, end
  in_1 : Inport  Orientation=left
  Constant : Constant  Orientation=left  Value=0
  Constant1 : Constant  Orientation=left
  Switch : Switch  Orientation=left  SaturateOnIntegerOverflow=on  InputSameDT=on
  Switch1 : Switch  Orientation=left  SaturateOnIntegerOverflow=on  InputSameDT=on
  inv. : Fcn  Orientation=left  Expr=1/u
  neg : Gain  Orientation=left  Gain=-1  SaturateOnIntegerOverflow=on
  out_1 : Outport  Orientation=left  InitialOutput=0
  wires:
  Constant1/1 -> Switch1/1
  in_1/1 -> Switch1/3, neg/1
  neg/1 -> Switch1/2, Switch/2
  Switch1/1 -> inv./1
  Switch/1 -> out_1/1
  inv./1 -> Switch/3
  Constant/1 -> Switch/1

== system vasastaden_sort/Sewage plant/Biological stage/Predenitri- fication/Nitrification/ denitrification/N-org to NH4 ==
  In1 : Inport  Orientation=down
  In2 : Inport  Orientation=down  Port=2
  C-tot : Fcn  Orientation=down  Expr=u(10)
  Ctot degr. : Fcn  Orientation=down  Expr=u(10)
  N-org : Fcn  Orientation=down  Expr=u(3)-u(4)-u(5)
  N-org degraded  to NH4 : Product  Orientation=down  SaturateOnIntegerOverflow=on  InputSameDT=on
  NH4 increased : MATLABFcn  Orientation=down  MATLABFcn=[zeros(3,1); u ; zeros(17,1)]  OutputDimensions=totnr
  Part of C-tot degraded : Product  Orientation=down  SaturateOnIntegerOverflow=on  InputSameDT=on
  if u>0 then 1/u else 0 : Subsystem  Orientation=down
      mask Display: disp('1/u')
  Out1 : Outport  Orientation=down  InitialOutput=0
  wires:
  Ctot degr./1 -> Part of C-tot degraded/1
  In1/1 -> Ctot degr./1
  C-tot/1 -> if u>0 then 1/u else 0/1(in_1)
  if u>0 then 1/u else 0/1(out_1) -> Part of C-tot degraded/2
  In2/1 -> C-tot/1, N-org/1
  N-org/1 -> N-org degraded  to NH4/2
  N-org degraded  to NH4/1 -> NH4 increased/1
  NH4 increased/1 -> Out1/1
  Part of C-tot degraded/1 -> N-org degraded  to NH4/1

== system vasastaden_sort/Separate Sewer System  (36)/Stormwater/Storm water/Add pollutants in rain/Initial loss/Count zeros ==
  In1 : Inport
  Constant13 : Constant  Value=0
  Constant8 : Constant
  Counter1 : Subsystem  TreatAsAtomicUnit=on
  Gain1 : Gain  Gain=-1  SaturateOnIntegerOverflow=on
  Memory1 : Memory
  if u== 0 then 1 else 1 : Switch  SaturateOnIntegerOverflow=on  InputSameDT=on
  Out1 : Outport
  wires:
  if u== 0 then 1 else 1/1 -> Counter1/Enable
  Counter1/1(Out1) -> Memory1/1
  Constant8/1 -> if u== 0 then 1 else 1/1
  Gain1/1 -> if u== 0 then 1 else 1/2
  Constant13/1 -> if u== 0 then 1 else 1/3
  In1/1 -> Gain1/1
  Memory1/1 -> Out1/1

== system vasastaden_sort/Separate Sewer System  (36)/Stormwater/Storm water/Rain -> Stormwater/other surfaces/ackumulation and wash-off ==
  rain [mm] : Inport
  pollutant [ug] : Inport  Port=2
  Demux1 : Demux  Outputs=[1 -1]
  Mux : Mux  Inputs=2
  Mux1 : Mux  Inputs=3
  Specify initial condition here : UnitDelay  Orientation=left  X0=othermax2
  Terminator : Terminator
  Unit Delay : UnitDelay  Orientation=left  X0=delayinit
  ackumulation Fcn1 : MATLABFcn  MATLABFcn=ackumulation  OutputDimensions=nr_ex_H2O
  deltaP : Scope
      settings: YMin=0  YMax=2250
  washoff Fcn : MATLABFcn  MATLABFcn=washoff  OutputDimensions=totnr
  pollutants [ug] : Outport
  wires:
  washoff Fcn/1 -> Demux1/1
  Demux1/2 -> deltaP/1, Unit Delay/1, pollutants [ug]/1
  Mux/1 -> washoff Fcn/1
  Unit Delay/1 -> Mux1/2
  Specify initial condition here/1 -> Mux1/3
  ackumulation Fcn1/1 -> Mux/2, Specify initial condition here/1
  Demux1/1 -> Terminator/1
  rain [mm]/1 -> Mux/1
  Mux1/1 -> ackumulation Fcn1/1
  pollutant [ug]/1 -> Mux1/1

== system vasastaden_sort/Separate Sewer System  (36)/Stormwater/Storm water/Rain -> Stormwater/other surfaces/dry deposition ==
  Product : Product  Inputs=*/  SaturateOnIntegerOverflow=on  InputSameDT=on
  Product1 : Product  SaturateOnIntegerOverflow=on  InputSameDT=on
  area m2 : Constant  Orientation=up  Value=othera2
  timesteps/yr : Constant  Value=365*24*sph
  torrdep ug/m2*yr : Constant  Value=drydep
  pollutants [ug] : Outport
  wires:
  area m2/1 -> Product1/2
  Product1/1 -> pollutants [ug]/1
  Product/1 -> Product1/1
  torrdep ug/m2*yr/1 -> Product/1
  timesteps/yr/1 -> Product/2

== system vasastaden_sort/Separate Sewer System  (36)/Stormwater/Storm water/Rain -> Stormwater/other surfaces/rain on other surfaces ==
  rain [mm] : Inport
  Product1 : Product  SaturateOnIntegerOverflow=on  InputSameDT=on
  area [m2] : Constant  Value=othera2
  mm->m : Gain  Gain=0.001  SaturateOnIntegerOverflow=on
  rain [m3] : Outport
  wires:
  mm->m/1 -> Product1/1
  rain [mm]/1 -> mm->m/1
  area [m2]/1 -> Product1/2
  Product1/1 -> rain [m3]/1

== system vasastaden_sort/Separate Sewer System  (36)/Stormwater/Storm water/Rain -> Stormwater/road surfaces/accumulation and wash-off ==
  rain [mm] : Inport
  pollutant [ug] : Inport  Port=2
  Demux1 : Demux  Outputs=[1 -1]
  Mux : Mux  Inputs=2
  Mux1 : Mux  Inputs=3
  Specify initial condition here : UnitDelay  Orientation=left  X0=roadaccmax2
  Unit Delay : UnitDelay  Orientation=left  X0=delayinit
  ackumulation Fcn1 : MATLABFcn  MATLABFcn=ackumulation  OutputDimensions=nr_ex_H2O
  washoff Fcn : MATLABFcn  MATLABFcn=washoff  OutputDimensions=totnr
  rain [mm]1 : Outport
  pollutants [ug] : Outport  Port=2
  wires:
  Demux1/1 -> rain [mm]1/1
  pollutant [ug]/1 -> Mux1/1
  ackumulation Fcn1/1 -> Specify initial condition here/1, Mux/2
  Specify initial condition here/1 -> Mux1/3
  Mux1/1 -> ackumulation Fcn1/1
  Unit Delay/1 -> Mux1/2
  Mux/1 -> washoff Fcn/1
  washoff Fcn/1 -> Demux1/1
  rain [mm]/1 -> Mux/1
  Demux1/2 -> Unit Delay/1, pollutants [ug]/1

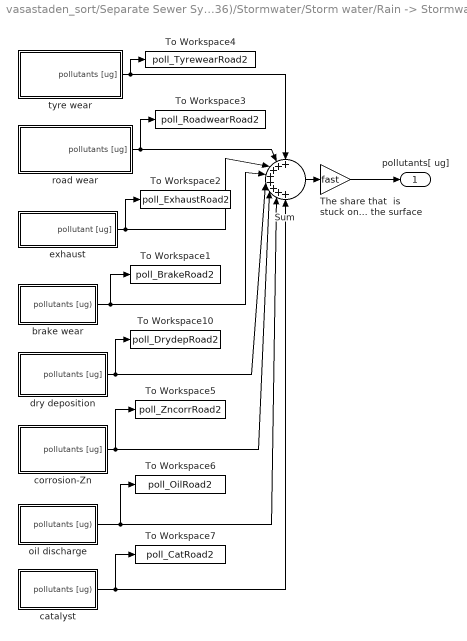
== system vasastaden_sort/Separate Sewer System  (36)/Stormwater/Storm water/Rain -> Stormwater/road surfaces/pollutants on roads ==
  Sum : Sum  Inputs=++++++++  SaturateOnIntegerOverflow=on  InputSameDT=on
  The share that  is stuck on the surface : Gain  Gain=fast  SaturateOnIntegerOverflow=on
  To Workspace1 : ToWorkspace  VariableName=poll_BrakeRoad2  SampleTime=-1  SaveFormat=Array
      settings: MaxDataPoints=1
  To Workspace10 : ToWorkspace  VariableName=poll_DrydepRoad2  SampleTime=-1  SaveFormat=Array
      settings: MaxDataPoints=1
  To Workspace2 : ToWorkspace  VariableName=poll_ExhaustRoad2  SampleTime=-1  SaveFormat=Array
      settings: MaxDataPoints=1
  To Workspace3 : ToWorkspace  VariableName=poll_RoadwearRoad2  SampleTime=-1  SaveFormat=Array
      settings: MaxDataPoints=1
  To Workspace4 : ToWorkspace  VariableName=poll_TyrewearRoad2  SampleTime=-1  SaveFormat=Array
      settings: MaxDataPoints=1
  To Workspace5 : ToWorkspace  VariableName=poll_ZncorrRoad2  SampleTime=-1  SaveFormat=Array
      settings: MaxDataPoints=1
  To Workspace6 : ToWorkspace  VariableName=poll_OilRoad2  SampleTime=-1  SaveFormat=Array
      settings: MaxDataPoints=1
  To Workspace7 : ToWorkspace  VariableName=poll_CatRoad2  SampleTime=-1  SaveFormat=Array
      settings: MaxDataPoints=1
  brake wear : Subsystem
  catalyst : Subsystem
  corrosion-Zn : Subsystem
  dry deposition : Subsystem
  exhaust : Subsystem
  oil discharge : Subsystem
  road wear : Subsystem
  tyre wear : Subsystem
  pollutants[ ug] : Outport
  wires:
  Sum/1 -> The share that  is stuck on the surface/1
  The share that  is stuck on the surface/1 -> pollutants[ ug]/1
  tyre wear/1(pollutants [ug]) -> Sum/1, To Workspace4/1
  road wear/1(pollutants [ug]) -> Sum/2, To Workspace3/1
  exhaust/1(pollutant [ug]) -> Sum/3, To Workspace2/1
  brake wear/1("pollutants [ug) ") -> Sum/4, To Workspace1/1
  dry deposition/1(pollutants [ug]) -> Sum/5, To Workspace10/1
  corrosion-Zn/1(pollutants [ug]) -> Sum/6, To Workspace5/1
  oil discharge/1("pollutants [ug) ") -> Sum/7, To Workspace6/1
  catalyst/1("pollutants [ug) ") -> Sum/8, To Workspace7/1

== system vasastaden_sort/Separate Sewer System  (36)/Stormwater/Storm water/Rain -> Stormwater/road surfaces/rain on road ==
  note: [m]
  rain [mm] : Inport
  pollutants [ug/m2] : Inport  Port=2
  Gain : Gain  Gain=0.001  SaturateOnIntegerOverflow=on
  Product : Product  SaturateOnIntegerOverflow=on  InputSameDT=on
  Product1 : Product  SaturateOnIntegerOverflow=on  InputSameDT=on
  area [m2] : Constant  Value=roada2
  rain [m3] : Outport
  pollutants [ug] : Outport  Port=2
  wires:
  Product1/1 -> pollutants [ug]/1
  pollutants [ug/m2]/1 -> Product1/2
  area [m2]/1 -> Product1/1, Product/2
  rain [mm]/1 -> Gain/1
  Gain/1 -> Product/1
  Product/1 -> rain [m3]/1

== system vasastaden_sort/Separate Sewer System  (36)/Stormwater/Storm water/Rain -> Stormwater/roofs/Pollutants on roofs ==
  Corrosion-Cu : Subsystem
  Corrosion-Zn : Subsystem
  Sum : Sum  Inputs=+++  SaturateOnIntegerOverflow=on  InputSameDT=on
  To Workspace10 : ToWorkspace  VariableName=poll_DrydepRoof2  SampleTime=-1  SaveFormat=Array
      settings: MaxDataPoints=1
  To Workspace11 : ToWorkspace  VariableName=poll_ZnRoof2  SampleTime=-1  SaveFormat=Array
      settings: MaxDataPoints=1
  To Workspace9 : ToWorkspace  VariableName=poll_CuRoof2  SampleTime=-1  SaveFormat=Array
      settings: MaxDataPoints=1
  dry deposition : Subsystem
  pollutants [ug] : Outport
  wires:
  Sum/1 -> pollutants [ug]/1
  Corrosion-Cu/1(pollutants [ug]) -> Sum/2, To Workspace9/1
  Corrosion-Zn/1(pollutants [ug]) -> Sum/3, To Workspace11/1
  dry deposition/1(pollutants [ug]) -> Sum/1, To Workspace10/1

== system vasastaden_sort/Separate Sewer System  (36)/Stormwater/Storm water/Rain -> Stormwater/roofs/ackumulation and wash-off ==
  rain [mm] : Inport
  pollutant [ug] : Inport  Port=2
  Demux1 : Demux  Outputs=[1 -1]
  Mux : Mux  Inputs=2
  Mux1 : Mux  Inputs=3
  Specify initial condition here : UnitDelay  Orientation=left  X0=roofmax2
  Terminator : Terminator
  Unit Delay : UnitDelay  Orientation=left  X0=delayinit
  ackumulation Fcn1 : MATLABFcn  MATLABFcn=ackumulation  OutputDimensions=nr_ex_H2O
  deltaP : Scope
      settings: TimeRange=50  YMin=0  YMax=1e+07
  washoff Fcn : MATLABFcn  MATLABFcn=washoff  OutputDimensions=totnr
  pollutants [ug] : Outport
  wires:
  Demux1/1 -> Terminator/1
  ackumulation Fcn1/1 -> Mux/2, Specify initial condition here/1
  Specify initial condition here/1 -> Mux1/3
  Unit Delay/1 -> Mux1/2
  Mux/1 -> washoff Fcn/1
  Demux1/2 -> pollutants [ug]/1, Unit Delay/1, deltaP/1
  washoff Fcn/1 -> Demux1/1
  Mux1/1 -> ackumulation Fcn1/1
  pollutant [ug]/1 -> Mux1/1
  rain [mm]/1 -> Mux/1

== system vasastaden_sort/Separate Sewer System  (36)/Stormwater/Storm water/Rain -> Stormwater/roofs/rain on roof surfaces ==
  rain [mm] : Inport
  Product1 : Product  SaturateOnIntegerOverflow=on  InputSameDT=on
  area [m2] : Constant  Value=roofa2
  mm->m : Gain  Gain=0.001  SaturateOnIntegerOverflow=on
  rain [m3] : Outport
  wires:
  Product1/1 -> rain [m3]/1
  area [m2]/1 -> Product1/2
  rain [mm]/1 -> mm->m/1
  mm->m/1 -> Product1/1

== system vasastaden_sort/Separate Sewer System  (36)/Stormwater/Storm water/Runoff/Subsystem1/if u>0 then u else 1 ==
  note: if u<=0, 0, else u, end
  in_1 : Inport
  Constant : Constant  Value=0
  Switch : Switch  SaturateOnIntegerOverflow=on  InputSameDT=on
  inv. : Fcn  Expr=u
  neg : Gain  Gain=-1  SaturateOnIntegerOverflow=on
  out_1 : Outport  InitialOutput=0
  wires:
  Switch/1 -> out_1/1
  Constant/1 -> Switch/1
  neg/1 -> Switch/2
  inv./1 -> Switch/3
  in_1/1 -> neg/1, inv./1

== system vasastaden_sort/Separate Sewer System  (36)/Stormwater/Storm water/Runoff (roads)/Subsystem1/if u>0 then u else 1 ==
  note: if u<=0, 0, else u, end
  in_1 : Inport
  Constant : Constant  Value=0
  Switch : Switch  SaturateOnIntegerOverflow=on  InputSameDT=on
  inv. : Fcn  Expr=u
  neg : Gain  Gain=-1  SaturateOnIntegerOverflow=on
  out_1 : Outport  InitialOutput=0
  wires:
  in_1/1 -> inv./1, neg/1
  inv./1 -> Switch/3
  neg/1 -> Switch/2
  Constant/1 -> Switch/1
  Switch/1 -> out_1/1

== system vasastaden_sort/Separate Sewer System  (1245)/Stormwater/Storm water/Add pollutants in rain/Initial loss/Count zeros ==
  In1 : Inport
  Constant13 : Constant  Value=0
  Constant8 : Constant
  Counter1 : Subsystem  TreatAsAtomicUnit=on
  Gain1 : Gain  Gain=-1  SaturateOnIntegerOverflow=on
  Memory1 : Memory
  if u== 0 then 1 else 1 : Switch  SaturateOnIntegerOverflow=on  InputSameDT=on
  Out1 : Outport
  wires:
  Memory1/1 -> Out1/1
  In1/1 -> Gain1/1
  Constant13/1 -> if u== 0 then 1 else 1/3
  Gain1/1 -> if u== 0 then 1 else 1/2
  Constant8/1 -> if u== 0 then 1 else 1/1
  Counter1/1(Out1) -> Memory1/1
  if u== 0 then 1 else 1/1 -> Counter1/Enable

== system vasastaden_sort/Separate Sewer System  (1245)/Stormwater/Storm water/Rain -> Stormwater/other surfaces/ackumulation and wash-off ==
  rain [mm] : Inport
  pollutant [ug] : Inport  Port=2
  Demux1 : Demux  Outputs=[1 -1]
  Mux : Mux  Inputs=2
  Mux1 : Mux  Inputs=3
  Specify initial condition here : UnitDelay  Orientation=left  X0=othermax
  Terminator : Terminator
  Unit Delay : UnitDelay  Orientation=left  X0=delayinit
  ackumulation Fcn1 : MATLABFcn  MATLABFcn=ackumulation  OutputDimensions=nr_ex_H2O
  deltaP : Scope
      settings: YMin=0  YMax=2250
  washoff Fcn : MATLABFcn  MATLABFcn=washoff  OutputDimensions=totnr
  pollutants [ug] : Outport
  wires:
  pollutant [ug]/1 -> Mux1/1
  Mux1/1 -> ackumulation Fcn1/1
  rain [mm]/1 -> Mux/1
  Demux1/1 -> Terminator/1
  ackumulation Fcn1/1 -> Specify initial condition here/1, Mux/2
  Specify initial condition here/1 -> Mux1/3
  Unit Delay/1 -> Mux1/2
  Mux/1 -> washoff Fcn/1
  Demux1/2 -> pollutants [ug]/1, Unit Delay/1, deltaP/1
  washoff Fcn/1 -> Demux1/1

== system vasastaden_sort/Separate Sewer System  (1245)/Stormwater/Storm water/Rain -> Stormwater/other surfaces/dry deposition ==
  Product : Product  Inputs=*/  SaturateOnIntegerOverflow=on  InputSameDT=on
  Product1 : Product  SaturateOnIntegerOverflow=on  InputSameDT=on
  area m2 : Constant  Orientation=up  Value=othera
  timesteps/yr : Constant  Value=365*24*sph
  torrdep ug/m2*yr : Constant  Value=drydep
  pollutants [ug] : Outport
  wires:
  timesteps/yr/1 -> Product/2
  torrdep ug/m2*yr/1 -> Product/1
  Product/1 -> Product1/1
  Product1/1 -> pollutants [ug]/1
  area m2/1 -> Product1/2

== system vasastaden_sort/Separate Sewer System  (1245)/Stormwater/Storm water/Rain -> Stormwater/other surfaces/rain on other surfaces ==
  rain [mm] : Inport
  Product1 : Product  SaturateOnIntegerOverflow=on  InputSameDT=on
  area [m2] : Constant  Value=othera
  mm->m : Gain  Gain=0.001  SaturateOnIntegerOverflow=on
  rain [m3] : Outport
  wires:
  Product1/1 -> rain [m3]/1
  area [m2]/1 -> Product1/2
  rain [mm]/1 -> mm->m/1
  mm->m/1 -> Product1/1

== system vasastaden_sort/Separate Sewer System  (1245)/Stormwater/Storm water/Rain -> Stormwater/road surfaces/accumulation and wash-off ==
  rain [mm] : Inport
  pollutant [ug] : Inport  Port=2
  Demux1 : Demux  Outputs=[1 -1]
  Mux : Mux  Inputs=2
  Mux1 : Mux  Inputs=3
  Specify initial condition here : UnitDelay  Orientation=left  X0=roadaccmax
  Unit Delay : UnitDelay  Orientation=left  X0=delayinit
  ackumulation Fcn1 : MATLABFcn  MATLABFcn=ackumulation  OutputDimensions=nr_ex_H2O
  washoff Fcn : MATLABFcn  MATLABFcn=washoff  OutputDimensions=totnr
  rain [mm]1 : Outport
  pollutants [ug] : Outport  Port=2
  wires:
  Demux1/2 -> pollutants [ug]/1, Unit Delay/1
  rain [mm]/1 -> Mux/1
  washoff Fcn/1 -> Demux1/1
  Mux/1 -> washoff Fcn/1
  Unit Delay/1 -> Mux1/2
  Mux1/1 -> ackumulation Fcn1/1
  Specify initial condition here/1 -> Mux1/3
  ackumulation Fcn1/1 -> Specify initial condition here/1, Mux/2
  pollutant [ug]/1 -> Mux1/1
  Demux1/1 -> rain [mm]1/1

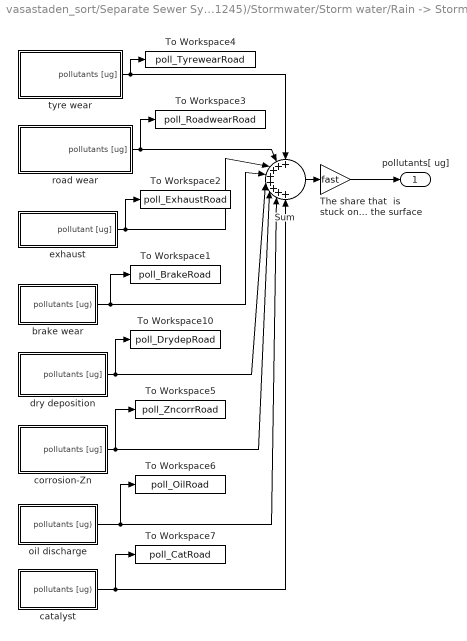
== system vasastaden_sort/Separate Sewer System  (1245)/Stormwater/Storm water/Rain -> Stormwater/road surfaces/pollutants on roads ==
  Sum : Sum  Inputs=++++++++  SaturateOnIntegerOverflow=on  InputSameDT=on
  The share that  is stuck on the surface : Gain  Gain=fast  SaturateOnIntegerOverflow=on
  To Workspace1 : ToWorkspace  VariableName=poll_BrakeRoad  SampleTime=-1  SaveFormat=Array
      settings: MaxDataPoints=1
  To Workspace10 : ToWorkspace  VariableName=poll_DrydepRoad  SampleTime=-1  SaveFormat=Array
      settings: MaxDataPoints=1
  To Workspace2 : ToWorkspace  VariableName=poll_ExhaustRoad  SampleTime=-1  SaveFormat=Array
      settings: MaxDataPoints=1
  To Workspace3 : ToWorkspace  VariableName=poll_RoadwearRoad  SampleTime=-1  SaveFormat=Array
      settings: MaxDataPoints=1
  To Workspace4 : ToWorkspace  VariableName=poll_TyrewearRoad  SampleTime=-1  SaveFormat=Array
      settings: MaxDataPoints=1
  To Workspace5 : ToWorkspace  VariableName=poll_ZncorrRoad  SampleTime=-1  SaveFormat=Array
      settings: MaxDataPoints=1
  To Workspace6 : ToWorkspace  VariableName=poll_OilRoad  SampleTime=-1  SaveFormat=Array
      settings: MaxDataPoints=1
  To Workspace7 : ToWorkspace  VariableName=poll_CatRoad  SampleTime=-1  SaveFormat=Array
      settings: MaxDataPoints=1
  brake wear : Subsystem
  catalyst : Subsystem
  corrosion-Zn : Subsystem
  dry deposition : Subsystem
  exhaust : Subsystem
  oil discharge : Subsystem
  road wear : Subsystem
  tyre wear : Subsystem
  pollutants[ ug] : Outport
  wires:
  catalyst/1("pollutants [ug) ") -> To Workspace7/1, Sum/8
  oil discharge/1("pollutants [ug) ") -> To Workspace6/1, Sum/7
  corrosion-Zn/1(pollutants [ug]) -> To Workspace5/1, Sum/6
  dry deposition/1(pollutants [ug]) -> To Workspace10/1, Sum/5
  brake wear/1("pollutants [ug) ") -> To Workspace1/1, Sum/4
  exhaust/1(pollutant [ug]) -> To Workspace2/1, Sum/3
  road wear/1(pollutants [ug]) -> To Workspace3/1, Sum/2
  tyre wear/1(pollutants [ug]) -> To Workspace4/1, Sum/1
  The share that  is stuck on the surface/1 -> pollutants[ ug]/1
  Sum/1 -> The share that  is stuck on the surface/1

== system vasastaden_sort/Separate Sewer System  (1245)/Stormwater/Storm water/Rain -> Stormwater/road surfaces/rain on road ==
  note: [m]
  rain [mm] : Inport
  pollutants [ug/m2] : Inport  Port=2
  Gain : Gain  Gain=0.001  SaturateOnIntegerOverflow=on
  Product : Product  SaturateOnIntegerOverflow=on  InputSameDT=on
  Product1 : Product  SaturateOnIntegerOverflow=on  InputSameDT=on
  area [m2] : Constant  Value=roada
  rain [m3] : Outport
  pollutants [ug] : Outport  Port=2
  wires:
  Product/1 -> rain [m3]/1
  Gain/1 -> Product/1
  rain [mm]/1 -> Gain/1
  area [m2]/1 -> Product/2, Product1/1
  pollutants [ug/m2]/1 -> Product1/2
  Product1/1 -> pollutants [ug]/1

== system vasastaden_sort/Separate Sewer System  (1245)/Stormwater/Storm water/Rain -> Stormwater/roofs/Pollutants on roofs ==
  Corrosion-Cu : Subsystem
  Corrosion-Zn : Subsystem
  Sum : Sum  Inputs=+++  SaturateOnIntegerOverflow=on  InputSameDT=on
  To Workspace10 : ToWorkspace  VariableName=poll_DrydepRoof  SampleTime=-1  SaveFormat=Array
      settings: MaxDataPoints=1
  To Workspace11 : ToWorkspace  VariableName=poll_ZnRoof  SampleTime=-1  SaveFormat=Array
      settings: MaxDataPoints=1
  To Workspace9 : ToWorkspace  VariableName=poll_CuRoof  SampleTime=-1  SaveFormat=Array
      settings: MaxDataPoints=1
  dry deposition : Subsystem
  pollutants [ug] : Outport
  wires:
  dry deposition/1(pollutants [ug]) -> To Workspace10/1, Sum/1
  Corrosion-Zn/1(pollutants [ug]) -> To Workspace11/1, Sum/3
  Corrosion-Cu/1(pollutants [ug]) -> To Workspace9/1, Sum/2
  Sum/1 -> pollutants [ug]/1

== system vasastaden_sort/Separate Sewer System  (1245)/Stormwater/Storm water/Rain -> Stormwater/roofs/ackumulation and wash-off ==
  rain [mm] : Inport
  pollutant [ug] : Inport  Port=2
  Demux1 : Demux  Outputs=[1 -1]
  Mux : Mux  Inputs=2
  Mux1 : Mux  Inputs=3
  Specify initial condition here : UnitDelay  Orientation=left  X0=roofmax
  Terminator : Terminator
  Unit Delay : UnitDelay  Orientation=left  X0=delayinit
  ackumulation Fcn1 : MATLABFcn  MATLABFcn=ackumulation  OutputDimensions=nr_ex_H2O
  deltaP : Scope
      settings: TimeRange=50  YMin=0  YMax=1e+07
  washoff Fcn : MATLABFcn  MATLABFcn=washoff  OutputDimensions=totnr
  pollutants [ug] : Outport
  wires:
  rain [mm]/1 -> Mux/1
  pollutant [ug]/1 -> Mux1/1
  Mux1/1 -> ackumulation Fcn1/1
  washoff Fcn/1 -> Demux1/1
  Demux1/2 -> deltaP/1, Unit Delay/1, pollutants [ug]/1
  Mux/1 -> washoff Fcn/1
  Unit Delay/1 -> Mux1/2
  Specify initial condition here/1 -> Mux1/3
  ackumulation Fcn1/1 -> Specify initial condition here/1, Mux/2
  Demux1/1 -> Terminator/1

== system vasastaden_sort/Separate Sewer System  (1245)/Stormwater/Storm water/Rain -> Stormwater/roofs/rain on roof surfaces ==
  rain [mm] : Inport
  Product1 : Product  SaturateOnIntegerOverflow=on  InputSameDT=on
  area [m2] : Constant  Value=roofa
  mm->m : Gain  Gain=0.001  SaturateOnIntegerOverflow=on
  rain [m3] : Outport
  wires:
  mm->m/1 -> Product1/1
  rain [mm]/1 -> mm->m/1
  area [m2]/1 -> Product1/2
  Product1/1 -> rain [m3]/1
